simulink subsystem "ModeloMovWilly"  (R2021b)
settings: Solver=VariableStepAuto  StartTime=0.0  StopTime=10.0  RelTol=1e-3
settings Model: Creator=yo  LastModifiedBy=yo

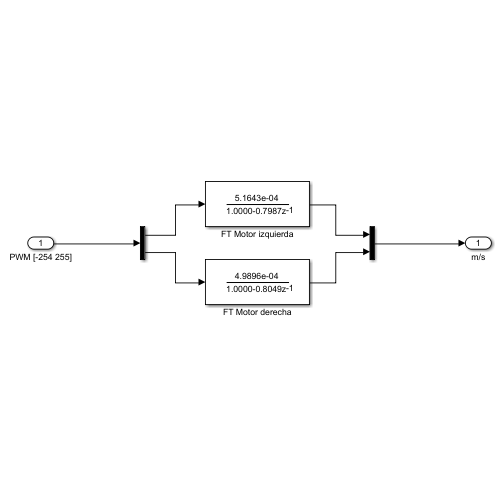
[thumbnail: Simulink's stored preview of the top-level diagram]
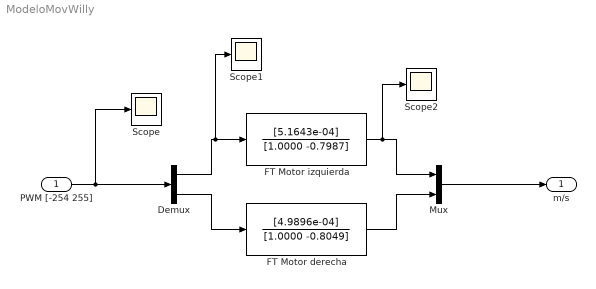
== system ModeloMovWilly ==
  PWM [-254 255] : Inport
  Demux : Demux  Outputs=2
  FT Motor derecha : DiscreteFilter  Numerator=[4.9896e-04]  Denominator=[1.0000 -0.8049]  SampleTime=0.01  OutDataTypeStr=int16
  FT Motor izquierda : DiscreteFilter  Numerator=[5.1643e-04]  Denominator=[1.0000 -0.7987]  SampleTime=0.01  OutDataTypeStr=int16
  Mux : Mux  Inputs=2
  Scope : Scope
  Scope1 : Scope
  Scope2 : Scope
  m/s : Outport
  wires:
  FT Motor izquierda/1 -> Mux/1, Scope2/1
  Demux/1 -> FT Motor izquierda/1, Scope1/1
  Demux/2 -> FT Motor derecha/1
  Mux/1 -> m/s/1
  FT Motor derecha/1 -> Mux/2
  PWM [-254 255]/1 -> Demux/1, Scope/1
